simulink model "MPC_Intersection_V2VandAIMandSTL"  (R2021b)
settings: Solver=ode45  StartTime=0.0  StopTime=50  RelTol=1e-3
model workspace (MAT data in the model file):
  firstWarning = 1
  originalScenarioChecksum = '44EB4239245A86A3DA7E3FEB76A9F5A7'
values from neighbouring files (symbols this model uses):
  curvature = (DX.*D2Y - DY.*D2X) ./(DX.^2+DY.^2).^(3/2)    [setUpModel_UScityblock2.m]
  direction = ones(length(gradbp),1)    [setUpModel_UScityblock2.m]
  gradbp = linspace(0,totalDistance,50)    [setUpModel_UScityblock2.m]
  psi_o = thetaRefab(1)*(pi/180)    [setUpModel_UScityblock2.m]
  speed_actor1_gdps = smooth(speedgradbpactor1,speedactor1le)    [velocity_profiles.m]
  speed_actor2_gdps = smooth(speedgradbpactor2,speedactor2le)    [velocity_profiles.m]
  speed_actor3_gdps = smooth(speedgradbpactor3,speedactor3le)    [velocity_profiles.m]
  speed_actor4_gdps = smooth(speedgradbpactor4,speedactor4le)    [velocity_profiles.m]
  speed_ego_gdps = smooth(speedgradbpego,speedegole)    [velocity_profiles.m]
  thetaRefab = zeros(length(gradbp),1)    [setUpModel_UScityblock2.m]
  x_gdps = smooth(gradbp,xwaypoints)    [setUpModel_UScityblock2.m]
  X_o = x_ego_i(1)    [setUpModel_UScityblock2.m]
  y_gdps = smooth(gradbp,ywaypoints)    [setUpModel_UScityblock2.m]
  Y_o = y_ego_i(1)    [setUpModel_UScityblock2.m]
undefined symbols (not defined in the file or in its folder): distancecovered, gradbpA1, gradbpA2, gradbpA3, gradbpA4, gradbpego, magnitude, n, q11, v2xCA
libraries: drivingscenarioandsensors x7, sim3dautolib x5, vehdynlibtirecommon x4, autolibutils x4, aerolibconvert2 x2, mpcadaslib x1, sim3dlib x1, simulink_extras x1, vehdynlibtire x1, simulink x1, autolibshared x1
(part 1 of 2)
settings Model: Creator=REHAN  LastModifiedBy=REHAN

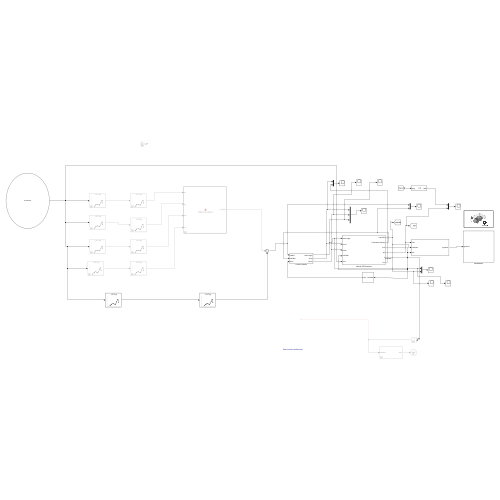
[thumbnail: Simulink's stored preview of the top-level diagram]
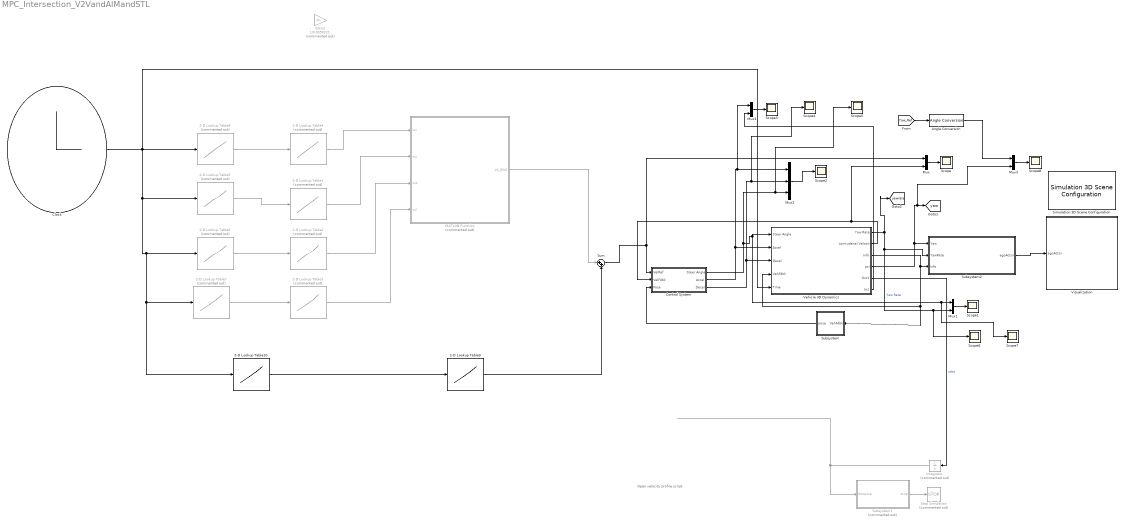
== system MPC_Intersection_V2VandAIMandSTL ==
  note: Open velocity profile script
  2-D Lookup Table1 : Lookup_n-D  Commented=on  NumberOfTableDimensions=1  BreakpointsForDimension1=gradbpA1  BreakpointsForDimension2=q11(:,2)  Table=speed_actor1_gdps  InterpMethod=Cubic spline  InternalRulePriority=Speed  RndMeth=Simplest  InputSameDT=on
  2-D Lookup Table10 : Lookup_n-D  NumberOfTableDimensions=1  BreakpointsForDimension1=n  BreakpointsForDimension2=q11(:,2)  Table=gradbpego  InterpMethod=Cubic spline  InternalRulePriority=Speed  RndMeth=Simplest  InputSameDT=on
  2-D Lookup Table2 : Lookup_n-D  Commented=on  NumberOfTableDimensions=1  BreakpointsForDimension1=gradbpA2  BreakpointsForDimension2=q11(:,2)  Table=speed_actor2_gdps  InterpMethod=Cubic spline  InternalRulePriority=Speed  RndMeth=Simplest  InputSameDT=on
  2-D Lookup Table3 : Lookup_n-D  Commented=on  NumberOfTableDimensions=1  BreakpointsForDimension1=gradbpA3  BreakpointsForDimension2=q11(:,2)  Table=speed_actor3_gdps  InterpMethod=Cubic spline  InternalRulePriority=Speed  RndMeth=Simplest  InputSameDT=on
  2-D Lookup Table4 : Lookup_n-D  Commented=on  NumberOfTableDimensions=1  BreakpointsForDimension1=gradbpA4  BreakpointsForDimension2=q11(:,2)  Table=speed_actor4_gdps  InterpMethod=Cubic spline  InternalRulePriority=Speed  RndMeth=Simplest  InputSameDT=on
  2-D Lookup Table5 : Lookup_n-D  Commented=on  NumberOfTableDimensions=1  BreakpointsForDimension1=n  BreakpointsForDimension2=q11(:,2)  Table=gradbpA1  InterpMethod=Cubic spline  InternalRulePriority=Speed  RndMeth=Simplest  InputSameDT=on
  2-D Lookup Table6 : Lookup_n-D  Commented=on  NumberOfTableDimensions=1  BreakpointsForDimension1=n  BreakpointsForDimension2=q11(:,2)  Table=gradbpA2  InterpMethod=Cubic spline  InternalRulePriority=Speed  RndMeth=Simplest  InputSameDT=on
  2-D Lookup Table7 : Lookup_n-D  Commented=on  NumberOfTableDimensions=1  BreakpointsForDimension1=n  BreakpointsForDimension2=q11(:,2)  Table=gradbpA3  InterpMethod=Cubic spline  InternalRulePriority=Speed  RndMeth=Simplest  InputSameDT=on
  2-D Lookup Table8 : Lookup_n-D  Commented=on  NumberOfTableDimensions=1  BreakpointsForDimension1=n  BreakpointsForDimension2=q11(:,2)  Table=gradbpA4  InterpMethod=Cubic spline  InternalRulePriority=Speed  RndMeth=Simplest  InputSameDT=on
  2-D Lookup Table9 : Lookup_n-D  NumberOfTableDimensions=1  BreakpointsForDimension1=gradbpego  BreakpointsForDimension2=q11(:,2)  Table=v2xCA  InterpMethod=Cubic spline  InternalRulePriority=Speed  RndMeth=Simplest  InputSameDT=on
  Angle Conversion : aerolibconvert2/Angle Conversion  IU=deg  OU=rad
  Clock : Clock
  Control System : Subsystem
  Gain2 : Gain  Commented=on  Gain=1/0.0058221
  Integrator : Integrator  Commented=on  InitialCondition=sqrt((X_o).^2+(Y_o).^2)
  MATLAB Function : MATLAB Function  Commented=on  TreatAsAtomicUnit=on
  Mux{,1,3..4} (4 alike) : Mux  Inputs=2
  Mux2 : Mux  Inputs=3
  Scope{,1..8} (9 alike) : Scope
  Simulation 3D Scene Configuration : sim3dlib/Simulation 3D Scene Configuration  Priority=0  ProjectFormat_internal=Default Scenes  ProjectFormat=Default Scenes  SceneDesc=US city block  ProjectName=C:\Program Files\MATLAB\R2021b\toolbox\shared\sim3d_projects\automotive_project\UE4\WindowsNoEditor\VehicleSimulation.exe  ScenePath=/Game/Maps/HwStrght  vehTagList={'Scene Origin';'SimulinkVehicle1';'SimulinkVehicle2';'SimulinkVehicle3';'SimulinkVehicle4';'SimulinkVehicle5'}  vehTag=SimulinkVehicle1  OpVisEn=off  Ts=1/60  EnableWindow=off  EnableWeather=off  SunAltitude=40.0  SunAzimuth=90  clouds=10  wind=1  fog=0  rain=79.0  sensorTag=MainCamera1  sensorId=1  sensorName=MainCamera1  mountLoc=Origin  offsetFlag=off  tmountOffset=[0, 0, 0]  rmountOffset=[0, 0, 0]  HorizontalResolution=1280  VerticalResolution=720  HorizontalFOV=60  mountPoint=[0 0 0]  mountOrientation=[0 0 0]  aMode=3  ID=1
      settings: SourceProductBaseCode=AE,DR,UV,VE
  Stop Simulation : Stop  Commented=on
  Subsystem : Subsystem
  Subsystem1 : Subsystem  Commented=on
  Subsystem2 : Subsystem
  Sum : Sum  Inputs=|++
  Vehicle 3D Dynamics : Subsystem
  "Visualization " : Subsystem
  tag scope: yaw=global, yawrate=global
  wires:
  Subsystem2/1(egoActor) -> "Visualization "/1(egoActor)
  Vehicle 3D Dynamics/3(Info) -> Subsystem/1(VehFdbk), Vehicle 3D Dynamics/4(VehFdbk), Subsystem2/3(Info)
  Vehicle 3D Dynamics/1(Yaw Rate) -> Scope6/1, Mux1/2, Subsystem2/2(YawRate), [yawrate]  "Yaw Rate"
  Vehicle 3D Dynamics/4(psi) -> Mux3/2, [yaw], Subsystem2/1(Yaw)
  Vehicle 3D Dynamics/2(Lonitudenal Velocity) -> Mux/2, Control System/2(VelFdbk)
  Subsystem/1(pose) -> Control System/3(Pose)
  Control System/2(Accel) -> Mux4/1, Mux2/1, Vehicle 3D Dynamics/2(Accel)
  Control System/3(Decel) -> Scope4/1, Mux2/2, Vehicle 3D Dynamics/3(Decel)
  Mux/1 -> Scope/1
  Mux1/1 -> Scope1/1
  Mux2/1 -> Scope2/1
  [Yaw_Ref] -> Angle Conversion/1
  Mux3/1 -> Scope8/1
  Integrator/1 -> Subsystem1/1(distance)
  Subsystem1/1(stop) -> Stop Simulation/1
  Vehicle 3D Dynamics/5(Out1) -> Integrator/1  "xdot"
  Angle Conversion/1 -> Mux3/1
  Vehicle 3D Dynamics/6(acc) -> Mux4/2
  Mux4/1 -> Scope3/1
  Sum/1 -> Mux/1, Control System/1(VelRef)
  2-D Lookup Table1/1 -> MATLAB Function/2(vxj)
  2-D Lookup Table2/1 -> MATLAB Function/3(vxk)
  2-D Lookup Table3/1 -> MATLAB Function/4(vxl)
  2-D Lookup Table4/1 -> MATLAB Function/1(vxi)
  2-D Lookup Table8/1 -> 2-D Lookup Table4/1
  2-D Lookup Table5/1 -> 2-D Lookup Table1/1
  2-D Lookup Table6/1 -> 2-D Lookup Table2/1
  2-D Lookup Table7/1 -> 2-D Lookup Table3/1
  Clock/1 -> Vehicle 3D Dynamics/5(Time), 2-D Lookup Table10/1, 2-D Lookup Table7/1, 2-D Lookup Table6/1, 2-D Lookup Table5/1, 2-D Lookup Table8/1
  MATLAB Function/1(VX_EGO) -> Sum/1
  2-D Lookup Table10/1 -> 2-D Lookup Table9/1
  2-D Lookup Table9/1 -> Sum/2
  Control System/1(Steer Angle) -> Scope5/1, Mux2/3, Scope7/1, Mux1/1, Vehicle 3D Dynamics/1(Steer Angle)

== system MPC_Intersection_V2VandAIMandSTL/Control System ==
  note: Controller
  VelRef : Inport
  VelFdbk : Inport  Port=2
  Pose : Inport  Port=3
  MPC Based Controller : Subsystem  VariantControl=Stanley
  Steer Angle : Outport
  Accel : Outport  Port=2
  Decel : Outport  Port=3
  wires:
  VelFdbk/1 -> MPC Based Controller/3(VelFdbk)
  Pose/1 -> MPC Based Controller/1(Pose)
  VelRef/1 -> MPC Based Controller/2(VelRef)
  MPC Based Controller/3(DecelCmd) -> Decel/1  "Decel"
  MPC Based Controller/2(AccelCmd) -> Accel/1  "Accel"
  MPC Based Controller/1(WheelSteeringAngle) -> Steer Angle/1  "Steer Angle"

== system MPC_Intersection_V2VandAIMandSTL/Subsystem ==
  VehFdbk : Inport
  Bus Selector : BusSelector  OutputSignals=InertFrm.Cg.Disp.X,InertFrm.Cg.Disp.Y,InertFrm.Cg.Ang.psi
  Gain1 : Gain  Gain=180/pi
  Mux : Mux  Inputs=3
  Transpose : Math  Operator=transpose  SignedPower=on  SaturateOnIntegerOverflow=on
  pose : Outport
  wires:
  Mux/1 -> Transpose/1
  VehFdbk/1 -> Bus Selector/1
  Bus Selector/1 -> Mux/1  "<X>"
  Gain1/1 -> Mux/3
  Bus Selector/2 -> Mux/2  "<Y>"
  Transpose/1 -> pose/1
  Bus Selector/3 -> Gain1/1  "<psi>"

== system MPC_Intersection_V2VandAIMandSTL/Subsystem1 ==
  distance : Inport
  Constant : Constant
  Constant3 : Constant  Value=0
  Switch : Switch  Threshold=distancecovered-10
  stop : Outport
  wires:
  Switch/1 -> stop/1
  Constant3/1 -> Switch/3
  distance/1 -> Switch/2
  Constant/1 -> Switch/1

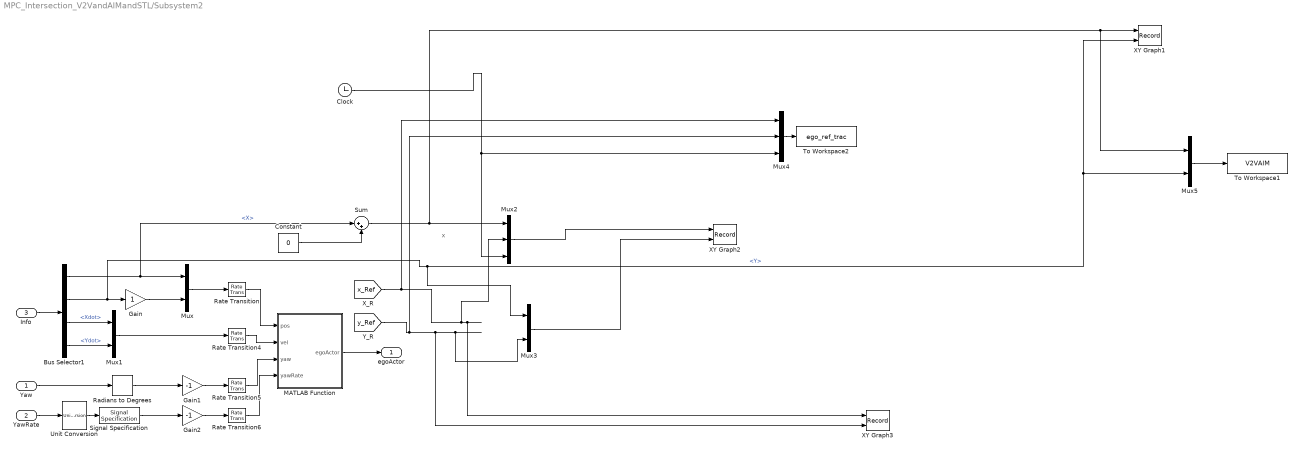
== system MPC_Intersection_V2VandAIMandSTL/Subsystem2 ==
  note: x
  Yaw : Inport
  YawRate : Inport  Port=2
  Info : Inport  Port=3
  Bus Selector1 : BusSelector  OutputSignals=InertFrm.Cg.Disp.X,InertFrm.Cg.Disp.Y,InertFrm.Cg.Vel.Xdot,InertFrm.Cg.Vel.Ydot
  Clock : Clock
  Constant : Constant  Value=0
  Gain : Gain
  Gain1 : Gain  Gain=-1
  Gain2 : Gain  Gain=-1
  MATLAB Function : MATLAB Function  TreatAsAtomicUnit=on
  Mux{,1,3,5} (4 alike) : Mux  Inputs=2
  Mux2 : Mux  Inputs=3
  Mux4 : Mux  Inputs=3
  Radians to Degrees : simulink_extras/Transformations/Radians to Degrees
  Rate Transition{,4..6} (4 alike) : RateTransition
  Signal Specification : SignalSpecification  Unit=deg/s
  Sum : Sum  Inputs=|++
  To Workspace1 : ToWorkspace  VariableName=V2VAIM  SaveFormat=Timeseries  SampleTime=-1
  To Workspace2 : ToWorkspace  VariableName=ego_ref_trac  SaveFormat=Timeseries  SampleTime=-1
  Unit Conversion : UnitConversion
  XY Graph1 : Record  FileSettingsInternal="{\"entries\":[{\"content\":{\"excelSettings\":{\"content\":{},\"type\":\"Streamout.ExcelSettings\"}},\"type\":\"Streamout.FileSettingStorage\",\"uuid\":\"2f12852f-246b-4ef9-8937-bb063900e442\"}],\"packageUris\":[\"http://schema.mathworks.com/mf0/streamout_blocks/R2020a\"],\"version\":\"1.0\"}"  Layout=[1 1]  SignalsInternal="{\"entries\":[{\"content\":{\"signals\":[{\"content\":{\"blockPath\":[\"MPC_Intersection_V2VandAIM/Subsystem2/XY Graph1\"],\"channel\":[],\"dimensions\":[1],\"domain\":\"MPC_Intersection_V2VandAIM/Subsystem2/XY Graph1\",\"lineColor\":\"#d95319\",\"plots\":[],\"port\":1,\"sid\":[\"\"],\"signalID\":357033,\"signalName\":\"Sum\"},\"type\":\"RecordBlkView.Signal\",\"uuid\":\"05f50db8-9dc6-4afe-ab3d-ad6a50919f12\"},{\"content\":{\"blockPath\":[\"MPC_Intersection_V2VandAIM/Subsystem2/XY Graph1\"],\"channel\":[],\"dimensions\":[1],\"domain\":\"MPC_Intersection_V2VandAIM/Subsystem2/XY Graph1\",\"lineColor\":\"#edb120\",\"plots\":[],\"port\":2,\"sid\":[\"\"],\"signalID\":357037,\"signalName\":\"<Y>\"},\"type\":\"RecordBlkView.Signal\",\"uuid\":\"f6264113-20c8-4f22-95b1-a6aed961d63f\"}]},\"type\":\"RecordBlkView.InputSignals\",\"uuid\":\"69c98a76-69b8-42fe-ae6b-722c9eef4afe\"}],\"packageUris\":[\"http://schema.mathworks.com/mf0/streamout_blocks/R2020a\"],\"version\":\"1.0\"}"  VisualizationBindings="{\"xyplotplugin\":{\"info\":[{\"series\":[],\"subplotID\":1}]}}"  CompatibilityTag=XY
  XY Graph2 : Record  FileSettingsInternal="{\"entries\":[{\"content\":{\"excelSettings\":{\"content\":{},\"type\":\"Streamout.ExcelSettings\"}},\"type\":\"Streamout.FileSettingStorage\",\"uuid\":\"6b49d13c-c461-41bf-8846-62c54b908676\"}],\"packageUris\":[\"http://schema.mathworks.com/mf0/streamout_blocks/R2020a\"],\"version\":\"1.0\"}"  Layout=[1 1]  SignalsInternal="{\"entries\":[{\"content\":{\"signals\":[{\"content\":{\"blockPath\":[\"MPC_Intersection_V2VandAIM/Subsystem2/XY Graph2\"],\"channel\":[],\"dimensions\":[3],\"domain\":\"MPC_Intersection_V2VandAIM/Subsystem2/XY Graph2\",\"hasChildren\":true,\"lineColor\":\"#7e2f8e\",\"plots\":[],\"port\":1,\"sid\":[\"\"],\"signalID\":357041,\"signalName\":\"Mux2\"},\"type\":\"RecordBlkView.Signal\",\"uuid\":\"150ad6de-05ca-4e16-9ea5-6f734c90b908\"},{\"content\":{\"blockPath\":[\"MPC_Intersection_V2VandAIM/Subsystem2/XY Graph2\"],\"channel\":[1],\"dimensions\":[3],\"domain\":\"MPC_Intersection_V2VandAIM/Subsystem2/XY Graph2\",\"lineColor\":\"#77ac30\",\"parentID\":357041,\"plots\":[],\"port\":1,\"sid\":[\"\"],\"signalID\":357042,\"signalName\":\"Mux2\"},\"type\":\"RecordBlkView.Signal\",\"uuid\":\"b4915db6-c8af-41c7-9b58-5548bd9cc9e2\"},{\"content\":{\"blockPath\":[\"MPC_Intersection_V2VandAIM/Subsystem2/XY Graph2\"],\"channel\":[],\"dimensions\":[2],\"domain\":\"MPC_Intersection_V2VandAIM/Subsystem2/XY Graph2\",\"hasChildren\":true,\"lineColor\":\"#4dbeee\",\"plots\":[],\"port\":2,\"sid\":[\"\"],\"signalID\":357046,\"signalName\":\"Mux3\"},\"type\":\"RecordBlkView.Signal\",\"uuid\":\"ee75895b-d730-4bf5-9f29-4dbf03fe07c6\"},{\"content\":{\"blockPath\":[\"MPC_Intersection_V2VandAIM/Subsystem2/XY Graph2\"],\"channel\":[1],\"dimensions\":[2],\"domain\":\"MPC_Intersection_V2VandAIM/Subsystem2/XY Graph2\",\"lineColor\":\"#a2142f\",\"parentID\":357046,\"plots\":[],\"port\":2,\"sid\":[\"\"],\"signalID\":357047,\"signalName\":\"Mux3\"},\"type\":\"RecordBlkView.Signal\",\"uuid\":\"339475a3-838f-4545-9489-51cd50d7a86b\"}]},\"type\":\"RecordBlkView.InputSignals\",\"uuid\":\"f0fde65e-7344-42f7-9758-ec72a1af721b\"}],\"packageUris\":[\"http://schema.mathworks.com/mf0/streamout_blocks/R2020a\"],\"version\":\"1.0\"}"  VisualizationBindings="{\"xyplotplugin\":{\"info\":[{\"series\":[],\"subplotID\":1}]}}"  CompatibilityTag=XY
  XY Graph3 : Record  FileSettingsInternal="{\"entries\":[{\"content\":{\"excelSettings\":{\"content\":{},\"type\":\"Streamout.ExcelSettings\"}},\"type\":\"Streamout.FileSettingStorage\",\"uuid\":\"24a241bf-8d8e-474c-b7bc-76b4d2e06980\"}],\"packageUris\":[\"http://schema.mathworks.com/mf0/streamout_blocks/R2020a\"],\"version\":\"1.0\"}"  Layout=[1 1]  SignalsInternal="{\"entries\":[{\"content\":{\"signals\":[{\"content\":{\"blockPath\":[\"MPC_Intersection_V2VandAIM/Subsystem2/XY Graph3\"],\"channel\":[],\"dimensions\":[1],\"domain\":\"MPC_Intersection_V2VandAIM/Subsystem2/XY Graph3\",\"lineColor\":\"#139fff\",\"plots\":[],\"port\":1,\"sid\":[\"\"],\"signalID\":357051,\"signalName\":\"X_R\"},\"type\":\"RecordBlkView.Signal\",\"uuid\":\"67cfc854-4ab1-4cce-b77a-7abc147af39a\"},{\"content\":{\"blockPath\":[\"MPC_Intersection_V2VandAIM/Subsystem2/XY Graph3\"],\"channel\":[],\"dimensions\":[1],\"domain\":\"MPC_Intersection_V2VandAIM/Subsystem2/XY Graph3\",\"lineColor\":\"#ff6929\",\"plots\":[],\"port\":2,\"sid\":[\"\"],\"signalID\":357055,\"signalName\":\"Y_R\"},\"type\":\"RecordBlkView.Signal\",\"uuid\":\"aa72a502-d578-4dc8-aeef-fdcf7ff26e0e\"}]},\"type\":\"RecordBlkView.InputSignals\",\"uuid\":\"33211d98-26d3-424d-a838-ac910746517b\"}],\"packageUris\":[\"http://schema.mathworks.com/mf0/streamout_blocks/R2020a\"],\"version\":\"1.0\"}"  VisualizationBindings="{\"xyplotplugin\":{\"info\":[{\"series\":[],\"subplotID\":1}]}}"  CompatibilityTag=XY
  egoActor : Outport
  wires:
  Mux/1 -> Rate Transition/1
  Rate Transition/1 -> MATLAB Function/1(pos)
  Rate Transition4/1 -> MATLAB Function/2(vel)
  Signal Specification/1 -> Gain2/1
  Bus Selector1/4 -> Mux1/2  "<Ydot>"
  Rate Transition5/1 -> MATLAB Function/3(yaw)
  Rate Transition6/1 -> MATLAB Function/4(yawRate)
  Bus Selector1/1 -> Sum/1, Mux/1  "<X>"
  Mux1/1 -> Rate Transition4/1
  YawRate/1 -> Unit Conversion/1
  Yaw/1 -> Radians to Degrees/1
  Radians to Degrees/1 -> Gain1/1
  Info/1 -> Bus Selector1/1
  Gain2/1 -> Rate Transition6/1
  Unit Conversion/1 -> Signal Specification/1
  Gain1/1 -> Rate Transition5/1
  Bus Selector1/3 -> Mux1/1  "<Xdot>"
  MATLAB Function/1(egoActor) -> egoActor/1
  [x_Ref] -> Mux4/1, Mux2/2, XY Graph3/1
  Gain/1 -> Mux/2
  [y_Ref] -> Mux4/2, XY Graph3/2, Mux3/2
  Mux2/1 -> XY Graph2/1
  Mux3/1 -> XY Graph2/2
  Bus Selector1/2 -> Mux3/1, XY Graph1/2, Mux5/2, Gain/1  "<Y>"
  Sum/1 -> XY Graph1/1, Mux5/1, Mux2/1
  Constant/1 -> Sum/2
  Clock/1 -> Mux4/3, Mux2/3
  Mux5/1 -> To Workspace1/1
  Mux4/1 -> To Workspace2/1

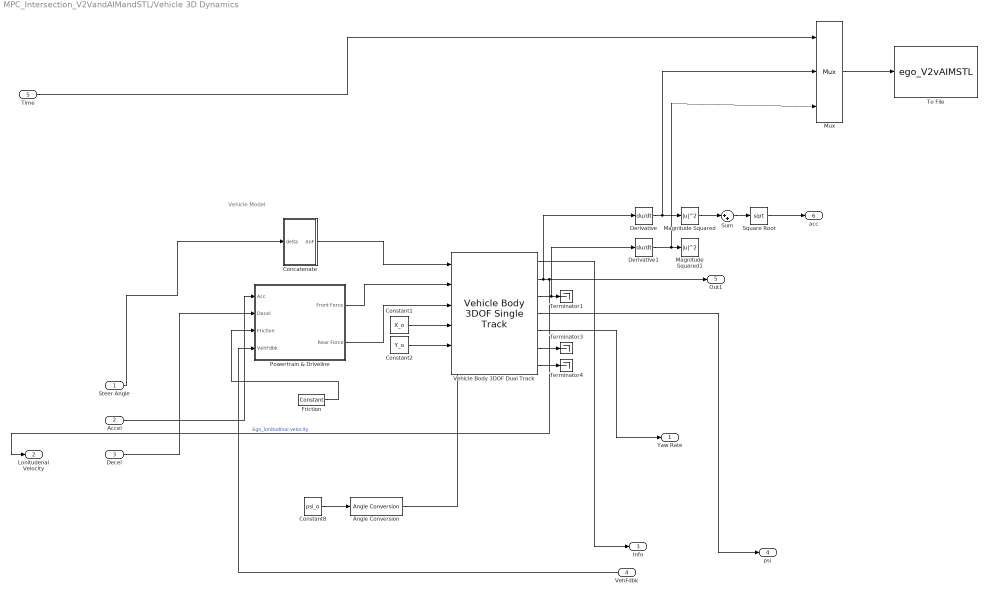
== system MPC_Intersection_V2VandAIMandSTL/Vehicle 3D Dynamics ==
  note: Vehicle Model
  Steer Angle : Inport
  Accel : Inport  Port=2
  Decel : Inport  Port=3
  VehFdbk : Inport  Port=4
  Time : Inport  Port=5
  Angle Conversion : aerolibconvert2/Angle Conversion  IU=rad  OU=deg
  Concatenate : Subsystem
  Constant1 : Constant  Value=X_o
  Constant2 : Constant  Value=Y_o
  Constant8 : Constant  Value=psi_o
  Derivative : Derivative
  Derivative1 : Derivative
  Friction : vehdynlibtirecommon/Constant  const=1  numWheels=4
      settings: SourceProductBaseCode=VE
  Magnitude Squared : Math  Operator=magnitude^2  SaturateOnIntegerOverflow=on
  Magnitude Squared1 : Math  Operator=magnitude^2  SaturateOnIntegerOverflow=on
  Mux : Mux  Inputs=3
  Powertrain & Driveline : Subsystem
      mask Display: image('vdbslibpt.png');
  Square Root : Sqrt  SaturateOnIntegerOverflow=on
  Sum : Sum  Inputs=|++
  Terminator1 : Terminator
  Terminator3 : Terminator
  Terminator4 : Terminator
  To File : ToFile  Filename=ego_V2vAIMSTL  MatrixName=waypointstimeseries
      settings: Decimation=100
  Vehicle Body 3DOF Dual Track : autolibshared/Vehicle Body 3DOF Single Track  trackMode=Dual  inputMode=External forces  frontSteerMode=on  rearSteerMode=off  windMode=off  muMode=off  extFMode=off  extMMode=off  htchFMode=off  htchMMode=off  extXo=on  extpsio=on  extxdoto=off  extro=off  extYo=on  extTamb=off  extydoto=off  aMode=2  NF=2  NR=2  m=2000  a=1.4  b=1.4  h=0.35  dh=1  hh=0.2  X_o=0  xdot_o=speed_ego_gdps(1)  CalphaMode=off  sigmaMode=on  d=0  hl=0  w=[1.4,1.4]  Cy_f=12e3  Cy_r=11e3  sigma_f=.1  sigma_r=.1  alpha_f_brk=[-.1 .1]  Cy_f_data=[-9e3 9e3]  alpha_r_brk=[-.1 .1]  Cy_r_data=[-9e3 9e3]  Y_o=0  ydot_o=0  Izz=1000  psi_o=0  r_o=0  Af=2  Cd=.3  Cl=.1  Cpm=.1  beta_w=[0:0.01:0.3]  Cs=[0:0.03:0.9]  Cym=[0:0.01:0.3]  Pabs=101325  Tair=273  g=9.81  mu=1  xdot_tol=.01  Fznom=5000  Fxtire_sat=7e4  Fytire_sat=7e4  longOff=0  latOff=0  vertOff=0  wrapAng=off
      settings: SourceProductBaseCode=PW,DR,MT,UV,VE
  Yaw Rate : Outport
  Lonitudenal Velocity : Outport  Port=2
  Info : Outport  Port=3
  psi : Outport  Port=4
  Out1 : Outport  Port=5
  acc : Outport  Port=6
  wires:
  Decel/1 -> Powertrain & Driveline/2(Decel)
  Constant8/1 -> Angle Conversion/1
  Vehicle Body 3DOF Dual Track/7 -> Terminator4/1
  Vehicle Body 3DOF Dual Track/1 -> Info/1
  Vehicle Body 3DOF Dual Track/6 -> Terminator3/1
  Constant2/1 -> Vehicle Body 3DOF Dual Track/5
  Friction/1 -> Powertrain & Driveline/3(Friction)
  Vehicle Body 3DOF Dual Track/2 -> Derivative/1, Out1/1, Lonitudenal Velocity/1  "Ego_lonitudinal velocity"
  Vehicle Body 3DOF Dual Track/3 -> Derivative1/1, Terminator1/1
  Constant1/1 -> Vehicle Body 3DOF Dual Track/4
  Accel/1 -> Powertrain & Driveline/1(Acc)
  Vehicle Body 3DOF Dual Track/5 -> Yaw Rate/1
  Vehicle Body 3DOF Dual Track/4 -> psi/1
  VehFdbk/1 -> Powertrain & Driveline/4(VehFdbk)
  Steer Angle/1 -> Concatenate/1(delta)
  Concatenate/1(AnF) -> Vehicle Body 3DOF Dual Track/1
  Angle Conversion/1 -> Vehicle Body 3DOF Dual Track/6
  Derivative/1 -> Mux/2, Magnitude Squared/1
  Derivative1/1 -> Mux/3, Magnitude Squared1/1
  Magnitude Squared/1 -> Sum/1
  Sum/1 -> Square Root/1
  Square Root/1 -> acc/1
  Time/1 -> Mux/1
  Mux/1 -> To File/1
  Powertrain & Driveline/1(Front Force) -> Vehicle Body 3DOF Dual Track/2
  Powertrain & Driveline/2(Rear Force) -> Vehicle Body 3DOF Dual Track/3

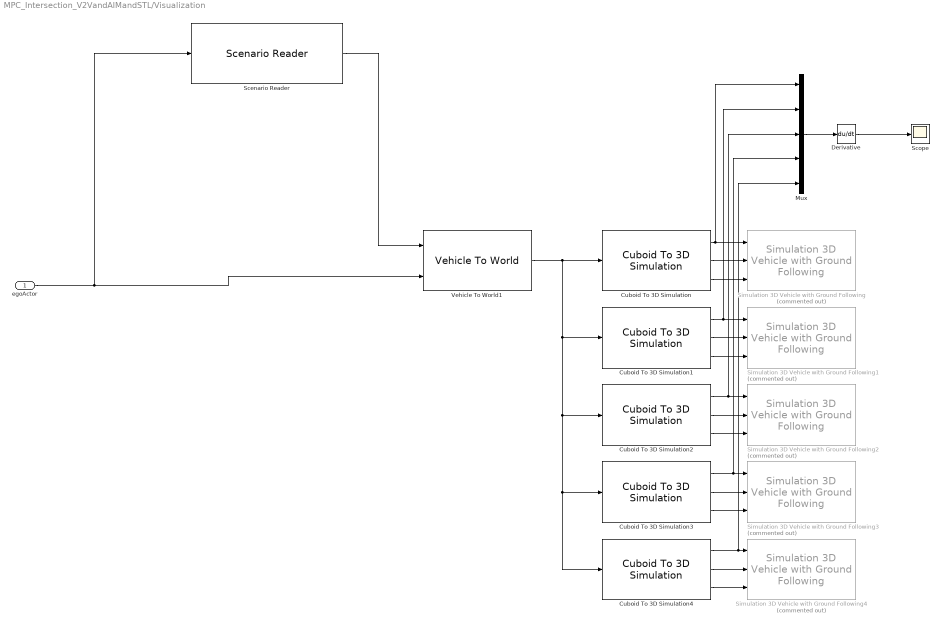
== system MPC_Intersection_V2VandAIMandSTL/Visualization  ==
  egoActor : Inport
  Cuboid To 3D Simulation : drivingscenarioandsensors/Cuboid To 3D Simulation  SpecifyActorID=off  ActorIDToConvert=1  SimulateUsing=Interpreted execution
      settings: SourceProductBaseCode=DR
  Cuboid To 3D Simulation1 : drivingscenarioandsensors/Cuboid To 3D Simulation  SpecifyActorID=off  ActorIDToConvert=2  SimulateUsing=Interpreted execution
      settings: SourceProductBaseCode=DR
  Cuboid To 3D Simulation2 : drivingscenarioandsensors/Cuboid To 3D Simulation  SpecifyActorID=off  ActorIDToConvert=3  SimulateUsing=Interpreted execution
      settings: SourceProductBaseCode=DR
  Cuboid To 3D Simulation3 : drivingscenarioandsensors/Cuboid To 3D Simulation  SpecifyActorID=off  ActorIDToConvert=4  SimulateUsing=Interpreted execution
      settings: SourceProductBaseCode=DR
  Cuboid To 3D Simulation4 : drivingscenarioandsensors/Cuboid To 3D Simulation  SpecifyActorID=off  ActorIDToConvert=4  SimulateUsing=Interpreted execution
      settings: SourceProductBaseCode=DR
  Derivative : Derivative
  Mux : Mux  Inputs=5
  Scenario Reader : drivingscenarioandsensors/Scenario Reader  ScenarioSource=From file  ScenarioFileName=C:\Users\REHAN\OneDrive - The Ohio State University\UTC PNT Resilience\simulation files\USCityBlock2.mat  ScenarioVariableName=scenario  OutputCoordinateSystem=Vehicle coordinates  EgoVehicleSource=Input port  EgoVehicleActorID=1  OrientVehiclesOnRoad=on  OutputEgoVehiclePose=on  OutputEgoVehicleState=off  SampleTime=0.1  LaneBoundaryOutput=None  LaneBoundaryDistance=0:0.5:9.5  LaneBoundaryLocation=Center of lane markings  BusNameSource=Auto  BusName=BusActors  BusNumActorsSource=Scenario  BusNumActors=100  BusName2Source=Auto  BusName2=BusLaneBoundaries  BusNumLaneBoundariesSource=Scenario  BusNumLaneBoundaries=10  BusName3Source=Auto  BusName3=BusEgoActor  BusName4Source=Auto  BusName4=BusEgoState  ShowCoordinateLabels=on  SimulateUsing=Interpreted execution
  Scope : Scope
  Simulation 3D Vehicle with Ground Following : sim3dautolib/Simulation 3D Vehicle with Ground Following  Priority=-1  Commented=on  PassVehMesh=Muscle car  PassVehMesh_Internal=Muscle car  MeshPath=/MathWorksSimulation/Vehicles/Muscle/Meshes/SK_MuscleCar.SK_MuscleCar  TrackWidth=1.9  WheelBase=3  WheelRadius=0.35  VehColor=Red  VehColor_Internal=Red  InitialPos=[-150.9000,-1.8000, 0]  InitialRot=[0, 0,0.6853]  ActorName=SimulinkVehicle1  SampleTime=-1  ActorType=SimulinkVehicle  ID=1  aMode=3  ActorTag=SimulinkVehicle1  CoordinateScheme=ISO  VehLightsControl=off  HeadlightColor=[ 1, 1, 1 ]  HighBeamIntensity=100000  LowBeamIntensity=60000  HighBeamConeAngle=70  LowBeamConeAngle=70  LeftHeadlightOrientation=[ 0, 0 ]  RightHeadlightOrientation=[ 0, 0 ]  BrakelightIntensity=500  ReverselightIntensity=500  SignallightIntensity=500  SignallightPeriod=1  SignalPulseWidth=50  TransformOutportEnabled=off
      settings: SourceProductBaseCode=AE,DR,UV,VE
  Simulation 3D Vehicle with Ground Following1 : sim3dautolib/Simulation 3D Vehicle with Ground Following  Priority=-1  Commented=on  PassVehMesh=Muscle car  PassVehMesh_Internal=Muscle car  MeshPath=/MathWorksSimulation/Vehicles/Muscle/Meshes/SK_MuscleCar.SK_MuscleCar  TrackWidth=1.9  WheelBase=3  WheelRadius=0.35  VehColor=Orange  VehColor_Internal=Orange  InitialPos=[-110.9713, -28.0022, 0]  InitialRot=[0, 0, 86.1785]  ActorName=SimulinkVehicle2  SampleTime=-1  ActorType=SimulinkVehicle  ID=2  aMode=3  ActorTag=SimulinkVehicle2  CoordinateScheme=ISO  VehLightsControl=off  HeadlightColor=[ 1, 1, 1 ]  HighBeamIntensity=100000  LowBeamIntensity=60000  HighBeamConeAngle=70  LowBeamConeAngle=70  LeftHeadlightOrientation=[ 0, 0 ]  RightHeadlightOrientation=[ 0, 0 ]  BrakelightIntensity=500  ReverselightIntensity=500  SignallightIntensity=500  SignallightPeriod=1  SignalPulseWidth=50  TransformOutportEnabled=off
      settings: SourceProductBaseCode=AE,DR,UV,VE
  Simulation 3D Vehicle with Ground Following2 : sim3dautolib/Simulation 3D Vehicle with Ground Following  Priority=-1  Commented=on  PassVehMesh=Muscle car  PassVehMesh_Internal=Muscle car  MeshPath=/MathWorksSimulation/Vehicles/Muscle/Meshes/SK_MuscleCar.SK_MuscleCar  TrackWidth=1.9  WheelBase=3  WheelRadius=0.35  VehColor=Green  VehColor_Internal=Green  InitialPos=[-84.2000, 2.50, 0]  InitialRot=[0, 0, 176.7404]  ActorName=SimulinkVehicle3  SampleTime=-1  ActorType=SimulinkVehicle  ID=3  aMode=3  ActorTag=SimulinkVehicle3  CoordinateScheme=ISO  VehLightsControl=off  HeadlightColor=[ 1, 1, 1 ]  HighBeamIntensity=100000  LowBeamIntensity=60000  HighBeamConeAngle=70  LowBeamConeAngle=70  LeftHeadlightOrientation=[ 0, 0 ]  RightHeadlightOrientation=[ 0, 0 ]  BrakelightIntensity=500  ReverselightIntensity=500  SignallightIntensity=500  SignallightPeriod=1  SignalPulseWidth=50  TransformOutportEnabled=off
      settings: SourceProductBaseCode=AE,DR,UV,VE
  Simulation 3D Vehicle with Ground Following3 : sim3dautolib/Simulation 3D Vehicle with Ground Following  Priority=-1  Commented=on  PassVehMesh=Muscle car  PassVehMesh_Internal=Muscle car  MeshPath=/MathWorksSimulation/Vehicles/Muscle/Meshes/SK_MuscleCar.SK_MuscleCar  TrackWidth=1.9  WheelBase=3  WheelRadius=0.35  VehColor=Blue  VehColor_Internal=Blue  InitialPos=[-114.9284, 33.7974, 0]  InitialRot=[0, 0, 84.2930]  ActorName=SimulinkVehicle4  SampleTime=-1  ActorType=SimulinkVehicle  ID=4  aMode=3  ActorTag=SimulinkVehicle4  CoordinateScheme=ISO  VehLightsControl=off  HeadlightColor=[ 1, 1, 1 ]  HighBeamIntensity=100000  LowBeamIntensity=60000  HighBeamConeAngle=70  LowBeamConeAngle=70  LeftHeadlightOrientation=[ 0, 0 ]  RightHeadlightOrientation=[ 0, 0 ]  BrakelightIntensity=500  ReverselightIntensity=500  SignallightIntensity=500  SignallightPeriod=1  SignalPulseWidth=50  TransformOutportEnabled=off
      settings: SourceProductBaseCode=AE,DR,UV,VE
  Simulation 3D Vehicle with Ground Following4 : sim3dautolib/Simulation 3D Vehicle with Ground Following  Priority=-1  Commented=on  PassVehMesh=Muscle car  PassVehMesh_Internal=Muscle car  MeshPath=/MathWorksSimulation/Vehicles/Muscle/Meshes/SK_MuscleCar.SK_MuscleCar  TrackWidth=1.9  WheelBase=3  WheelRadius=0.35  VehColor=Red  VehColor_Internal=Red  InitialPos=[X_o, Y_o, 0]  InitialRot=[0, 0, psi_o]  ActorName=SimulinkVehicle5  SampleTime=-1  ActorType=SimulinkVehicle  ID=5  aMode=3  ActorTag=SimulinkVehicle5  CoordinateScheme=ISO  VehLightsControl=off  HeadlightColor=[ 1, 1, 1 ]  HighBeamIntensity=100000  LowBeamIntensity=60000  HighBeamConeAngle=70  LowBeamConeAngle=70  LeftHeadlightOrientation=[ 0, 0 ]  RightHeadlightOrientation=[ 0, 0 ]  BrakelightIntensity=500  ReverselightIntensity=500  SignallightIntensity=500  SignallightPeriod=1  SignalPulseWidth=50  TransformOutportEnabled=off
      settings: SourceProductBaseCode=AE,DR,UV,VE
  Vehicle To World1 : drivingscenarioandsensors/Vehicle To World  BusNameSource=Auto  BusName=BusVehicleToWorldActors  SimulateUsing=Interpreted execution
      settings: SourceProductBaseCode=DR
  wires:
  Cuboid To 3D Simulation2/3 -> Simulation 3D Vehicle with Ground Following2/3
  Cuboid To 3D Simulation/3 -> Simulation 3D Vehicle with Ground Following/3
  Vehicle To World1/1 -> Cuboid To 3D Simulation4/1, Cuboid To 3D Simulation3/1, Cuboid To 3D Simulation2/1, Cuboid To 3D Simulation1/1, Cuboid To 3D Simulation/1
  Cuboid To 3D Simulation2/1 -> Mux/3, Simulation 3D Vehicle with Ground Following2/1
  Cuboid To 3D Simulation/2 -> Simulation 3D Vehicle with Ground Following/2
  Cuboid To 3D Simulation/1 -> Mux/1, Simulation 3D Vehicle with Ground Following/1
  Cuboid To 3D Simulation2/2 -> Simulation 3D Vehicle with Ground Following2/2
  Cuboid To 3D Simulation3/2 -> Simulation 3D Vehicle with Ground Following3/2
  Cuboid To 3D Simulation3/1 -> Mux/4, Simulation 3D Vehicle with Ground Following3/1
  Cuboid To 3D Simulation3/3 -> Simulation 3D Vehicle with Ground Following3/3
  Cuboid To 3D Simulation1/3 -> Simulation 3D Vehicle with Ground Following1/3
  Cuboid To 3D Simulation1/1 -> Mux/2, Simulation 3D Vehicle with Ground Following1/1
  Cuboid To 3D Simulation1/2 -> Simulation 3D Vehicle with Ground Following1/2
  Cuboid To 3D Simulation4/1 -> Mux/5, Simulation 3D Vehicle with Ground Following4/1
  Cuboid To 3D Simulation4/2 -> Simulation 3D Vehicle with Ground Following4/2
  Cuboid To 3D Simulation4/3 -> Simulation 3D Vehicle with Ground Following4/3
  Scenario Reader/1 -> Vehicle To World1/1
  egoActor/1 -> Scenario Reader/1, Vehicle To World1/2
  Derivative/1 -> Scope/1
  Mux/1 -> Derivative/1

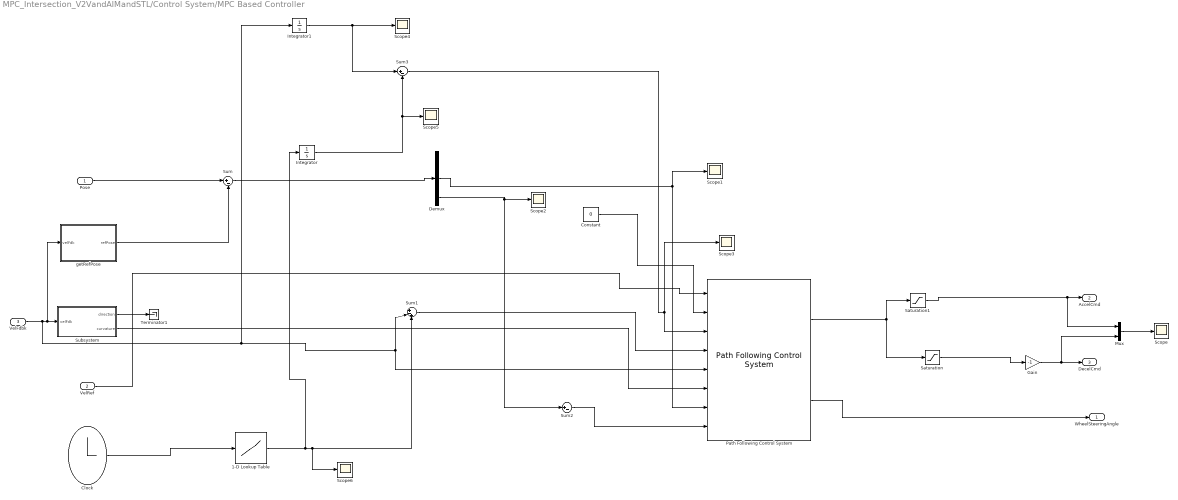
== system MPC_Intersection_V2VandAIMandSTL/Control System/MPC Based Controller ==
  Pose : Inport
  VelRef : Inport  Port=2
  VelFdbk : Inport  Port=3
  1-D Lookup Table : Lookup_n-D  NumberOfTableDimensions=1  BreakpointsForDimension1=n  Table=speed_actor4_gdps  InternalRulePriority=Speed  RndMeth=Simplest  InputSameDT=on
  Clock : Clock
  Constant : Constant  Value=0
  Demux : Demux  Outputs=3
  Gain : Gain  Gain=-1
  Integrator : Integrator
  Integrator1 : Integrator
  Mux : Mux  Inputs=2
  Path Following Control System : mpcadaslib/Path Following Control System  VariantControl=Variant2  ModelType=Use vehicle parameters  VehicleMass=1575  VehicleYawInertia=2875  LengthToFront=1.2  LengthToRear=1.6  FrontTireStiffness=19000  RearTireStiffness=33000  AccelTimeConstant=0.5  EgoModelMatrixA=[-2,zeros(1,3);1,zeros(1,3);zeros(1,2),-4.4021,-12.4603;zeros(1,2),1.3913,-5.1868]  EgoModelMatrixB=[2,zeros(1,3);zeros(1,2),24.1270,15.8609]'  EgoModelMatrixC=[zeros(3,1),eye(3)]  InitialLongVel=1  TransportLag=0  spaceCtrl=on  DefaultSpacing=0  MinSteering=-0.86  umin_ext=off  MaxSteering=0.86  umax_ext=off  MinAcceleration=-0.86  amin_ext=off  MaxAcceleration=0.86  amax_ext=off  Ts=0.1  PredictionHorizon=50  ControlHorizon=2  LongWeight=5000  LateralWeight=0.01  AccelRateWeight=3  SteerRateWeight=20  suboptimal=off  maxiter=10  datatypeopt=double  optmode=off  trackmode=off
      settings: SourceProductBaseCode=MP
  Saturation : Saturate  UpperLimit=0  LowerLimit=-3
  Saturation1 : Saturate  UpperLimit=3  LowerLimit=0
  Scope{,1..6} (7 alike) : Scope
  Subsystem : Subsystem
  Sum : Sum  Inputs=|+-
  Sum1 : Sum  Inputs=|+-+
  Sum2 : Sum  Inputs=|+-
  Sum3 : Sum  Inputs=|+-
  Terminator1 : Terminator
  getRefPose : Subsystem
  WheelSteeringAngle : Outport
  AccelCmd : Outport  Port=2
  DecelCmd : Outport  Port=3
  wires:
  VelFdbk/1 -> Integrator1/1, Path Following Control System/5, Sum1/2, Subsystem/1(velFdk), getRefPose/1(velFdk)
  getRefPose/1(refPose) -> Sum/2
  Subsystem/2(curvature) -> Path Following Control System/6
  Constant/1 -> Path Following Control System/2
  Path Following Control System/2 -> WheelSteeringAngle/1
  Path Following Control System/1 -> Saturation1/1, Saturation/1
  Saturation/1 -> Gain/1
  Mux/1 -> Scope/1
  Gain/1 -> Mux/2, DecelCmd/1
  Demux/2 -> Scope1/1, Path Following Control System/7
  Pose/1 -> Sum/1
  Subsystem/1(direction) -> Terminator1/1
  Saturation1/1 -> Mux/1, AccelCmd/1
  Sum/1 -> Demux/1
  Sum1/1 -> Path Following Control System/4
  Sum2/1 -> Path Following Control System/8
  Demux/3 -> Scope2/1, Sum2/1
  1-D Lookup Table/1 -> Integrator/1, Scope6/1, Sum1/3
  Clock/1 -> 1-D Lookup Table/1
  Sum3/1 -> Scope3/1, Path Following Control System/3
  Integrator1/1 -> Scope4/1, Sum3/1
  Integrator/1 -> Scope5/1, Sum3/2
  VelRef/1 -> Path Following Control System/1

== system MPC_Intersection_V2VandAIMandSTL/Vehicle 3D Dynamics/Concatenate ==
  delta : Inport
  Matrix Concatenate : Concatenate
  AnF : Outport  VectorParamsAs1DForOutWhenUnconnected=off
  tag scope: AnL=global, AnR=global
  wires:
  Matrix Concatenate/1 -> AnF/1
  delta/1 -> [AnR], Matrix Concatenate/2, Matrix Concatenate/1, [AnL]

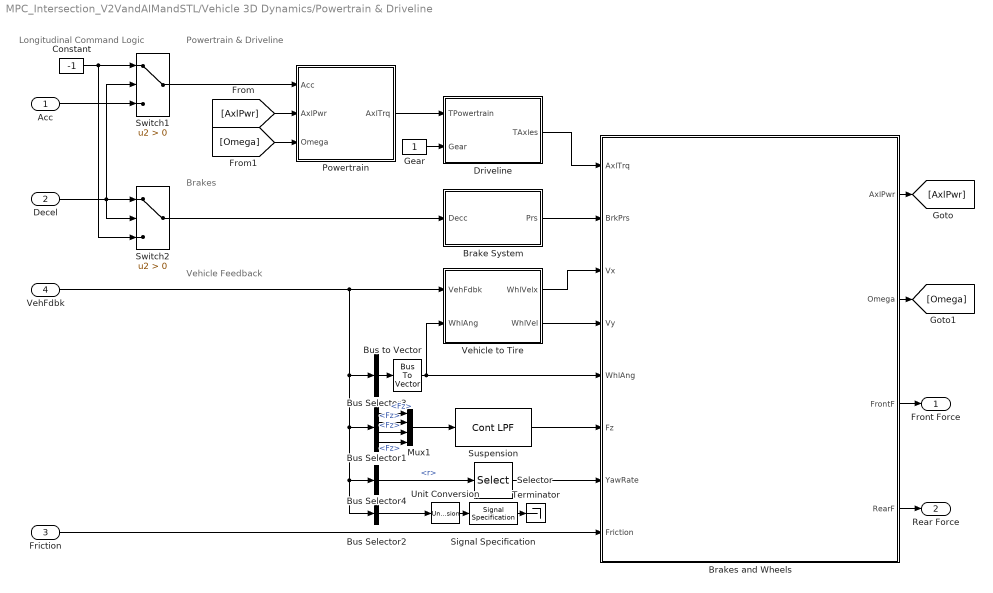
== system MPC_Intersection_V2VandAIMandSTL/Vehicle 3D Dynamics/Powertrain & Driveline ==
  note: Vehicle Feedback
  note: Powertrain & Driveline
  note: Brakes
  note: Longitudinal Command Logic
  Acc : Inport
  Decel : Inport  Port=2
  Friction : Inport  Port=3
  VehFdbk : Inport  Port=4
  Brake System : Subsystem
  Brakes and Wheels : Subsystem  TreatAsAtomicUnit=on
      mask Display: image('vdbslibwhls.png');
  Bus Selector1 : BusSelector  OutputSignals=BdyFrm.Forces.Tires.FrntTires.Lft.Fz,BdyFrm.Forces.Tires.FrntTires.Rght.Fz,BdyFrm.Forces.Tires.RearTires.Lft.Fz,BdyFrm.Forces.Tires.RearTires.Rght.Fz
  Bus Selector2 : BusSelector  OutputSignals=BdyFrm.Cg.Vel.xdot  OutputAsBus=on
  Bus Selector3 : BusSelector  OutputSignals=BdyFrm.FrntAxl.Steer.WhlAngFL,BdyFrm.FrntAxl.Steer.WhlAngFR,BdyFrm.RearAxl.Steer.WhlAngRL,BdyFrm.RearAxl.Steer.WhlAngRR  OutputAsBus=on
  Bus Selector4 : BusSelector  OutputSignals=BdyFrm.Cg.AngVel.r
  Bus to Vector : BusToVector
  Constant : Constant  Value=-1
  Driveline : Subsystem  Variant=on  VariantControlMode=label  VariantControl=Variant1  LabelModeActiveChoice=0
  Gear : Constant
  Mux1 : Mux
  Powertrain : Subsystem
  Selector : Selector  InputPortWidth=1  IndexOptions=Index vector (dialog)  Indices=[1 1 1 1]  OutputSizes=1
  Signal Specification : SignalSpecification  Unit=km/hr
  Suspension : autolibutils/Cont LPF  wc=10*pi*2  aMode=2
      settings: SourceProductBaseCode=PW,DR,MT,UV,VE
  Switch1 : Switch  Criteria=u2 > Threshold
  Switch2 : Switch  Criteria=u2 > Threshold
  Terminator : Terminator
  Unit Conversion : UnitConversion
  Vehicle to Tire : Subsystem
  Front Force : Outport  VectorParamsAs1DForOutWhenUnconnected=off
  Rear Force : Outport  Port=2  VectorParamsAs1DForOutWhenUnconnected=off
  wires:
  Vehicle to Tire/2(WhlVel) -> Brakes and Wheels/4(Vy)
  Vehicle to Tire/1(WhlVelx) -> Brakes and Wheels/3(Vx)
  Brakes and Wheels/1(AxlPwr) -> [AxlPwr]
  Brakes and Wheels/4(RearF) -> Rear Force/1
  Brakes and Wheels/3(FrontF) -> Front Force/1
  Brakes and Wheels/2(Omega) -> [Omega]
  VehFdbk/1 -> Vehicle to Tire/1(VehFdbk), Bus Selector3/1, Bus Selector1/1, Bus Selector4/1, Bus Selector2/1
  Selector/1 -> Brakes and Wheels/7(YawRate)
  Bus Selector4/1 -> Selector/1  "<r>"
  Friction/1 -> Brakes and Wheels/8(Friction)
  Gear/1 -> Driveline/2(Gear)
  Signal Specification/1 -> Terminator/1
  Unit Conversion/1 -> Signal Specification/1
  Bus Selector2/1 -> Unit Conversion/1
  Brake System/1(Prs) -> Brakes and Wheels/2(BrkPrs)
  Switch2/1 -> Brake System/1(Decc)
  [Omega] -> Powertrain/3(Omega)
  [AxlPwr] -> Powertrain/2(AxlPwr)
  Powertrain/1(AxlTrq) -> Driveline/1(TPowertrain)
  Switch1/1 -> Powertrain/1(Acc)
  Bus Selector1/4 -> Mux1/4  "<Fz>"
  Bus Selector1/3 -> Mux1/3  "<Fz>"
  Bus Selector1/2 -> Mux1/2  "<Fz>"
  Bus Selector1/1 -> Mux1/1  "<Fz>"
  Suspension/1 -> Brakes and Wheels/6(Fz)
  Mux1/1 -> Suspension/1
  Bus to Vector/1 -> Brakes and Wheels/5(WhlAng), Vehicle to Tire/2(WhlAng)
  Bus Selector3/1 -> Bus to Vector/1
  Driveline/1(TAxles) -> Brakes and Wheels/1(AxlTrq)
  Constant/1 -> Switch1/1, Switch2/3
  Acc/1 -> Switch1/3
  Decel/1 -> Switch2/1, Switch2/2, Switch1/2

== system MPC_Intersection_V2VandAIMandSTL/Control System/MPC Based Controller/Subsystem ==
  velFdk : Inport
  Curvature : Lookup_n-D  NumberOfTableDimensions=1  BreakpointsForDimension1=gradbp  Table=curvature  InternalRulePriority=Speed  RndMeth=Simplest  InputSameDT=on
  Direction : Lookup_n-D  NumberOfTableDimensions=1  BreakpointsForDimension1=gradbp  Table=direction  InternalRulePriority=Speed  RndMeth=Simplest  InputSameDT=on
  Integrator1 : Integrator
  direction : Outport
  curvature : Outport  Port=2
  wires:
  velFdk/1 -> Integrator1/1
  Integrator1/1 -> Direction/1, Curvature/1
  Curvature/1 -> curvature/1
  Direction/1 -> direction/1

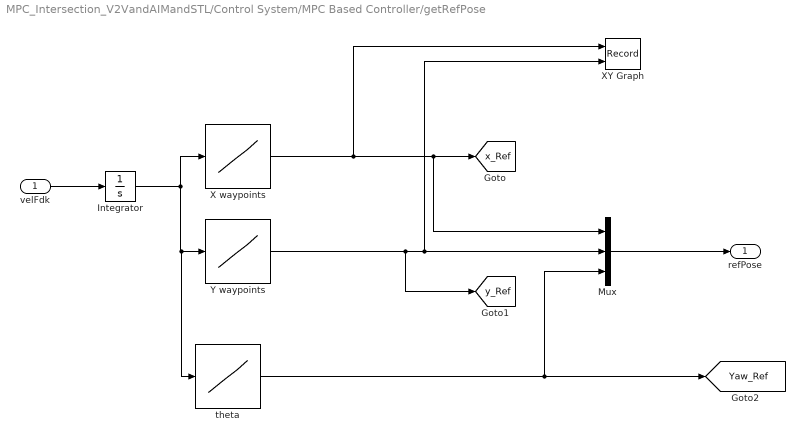
== system MPC_Intersection_V2VandAIMandSTL/Control System/MPC Based Controller/getRefPose ==
  velFdk : Inport
  Integrator : Integrator
  Mux : Mux  Inputs=3
  X waypoints : Lookup_n-D  NumberOfTableDimensions=1  BreakpointsForDimension1=gradbp  Table=x_gdps  InternalRulePriority=Speed  RndMeth=Simplest  InputSameDT=on
  XY Graph : Record  FileSettingsInternal="{\"entries\":[{\"content\":{\"excelSettings\":{\"content\":{},\"type\":\"Streamout.ExcelSettings\"}},\"type\":\"Streamout.FileSettingStorage\",\"uuid\":\"6aa8ae91-f7ce-496f-92bb-696a5a705436\"}],\"packageUris\":[\"http://schema.mathworks.com/mf0/streamout_blocks/R2020a\"],\"version\":\"1.0\"}"  Layout=[1 1]  SignalsInternal="{\"entries\":[{\"content\":{\"signals\":[{\"content\":{\"blockPath\":[\"MPC_Intersection_V2VandAIM/Control System/MPC Based Controller/getRefPose/XY Graph\"],\"channel\":[],\"dimensions\":[1],\"domain\":\"MPC_Intersection_V2VandAIM/Control System/MPC Based Controller/getRefPose/XY Graph\",\"lineColor\":\"#22b573\",\"plots\":[],\"port\":1,\"sid\":[\"\"],\"signalID\":357025,\"signalName\":\"X waypoints\"},\"type\":\"RecordBlkView.Signal\",\"uuid\":\"165d2a0c-33ff-47a3-a9f6-a99102be3ac1\"},{\"content\":{\"blockPath\":[\"MPC_Intersection_V2VandAIM/Control System/MPC Based Controller/getRefPose/XY Graph\"],\"channel\":[],\"dimensions\":[1],\"domain\":\"MPC_Intersection_V2VandAIM/Control System/MPC Based Controller/getRefPose/XY Graph\",\"lineColor\":\"#0072bd\",\"plots\":[],\"port\":2,\"sid\":[\"\"],\"signalID\":357029,\"signalName\":\"Y waypoints\"},\"type\":\"RecordBlkView.Signal\",\"uuid\":\"55140c9b-f205-4a31-9971-9d327590276e\"}]},\"type\":\"RecordBlkView.InputSignals\",\"uuid\":\"8cef2a80-f974-474f-9630-9d0ec5a192ec\"}],\"packageUris\":[\"http://schema.mathworks.com/mf0/streamout_blocks/R2020a\"],\"version\":\"1.0\"}"  VisualizationBindings="{\"xyplotplugin\":{\"info\":[{\"series\":[],\"subplotID\":1}]}}"  CompatibilityTag=XY
  Y waypoints : Lookup_n-D  NumberOfTableDimensions=1  BreakpointsForDimension1=gradbp  Table=y_gdps  InternalRulePriority=Speed  RndMeth=Simplest  InputSameDT=on
  theta : Lookup_n-D  NumberOfTableDimensions=1  BreakpointsForDimension1=gradbp  Table=thetaRefab  InternalRulePriority=Speed  RndMeth=Simplest  InputSameDT=on
  refPose : Outport
  tag scope: Yaw_Ref=global, x_Ref=global, y_Ref=global
  wires:
  Integrator/1 -> X waypoints/1, theta/1, Y waypoints/1
  velFdk/1 -> Integrator/1
  Mux/1 -> refPose/1
  X waypoints/1 -> XY Graph/1, [x_Ref], Mux/1
  Y waypoints/1 -> [y_Ref], XY Graph/2, Mux/2
  theta/1 -> Mux/3, [Yaw_Ref]

== system MPC_Intersection_V2VandAIMandSTL/Vehicle 3D Dynamics/Powertrain & Driveline/Brake System ==
  Decc : Inport
  Hydraulics : autolibutils/Cont LPF  wc=30*pi*2  aMode=2
      settings: SourceProductBaseCode=PW,DR,MT,UV,VE
  Pressure : Gain  Gain=15e7
  Saturation1 : Saturate  UpperLimit=inf  LowerLimit=0  ZeroCross=off
  Selector : Selector  InputPortWidth=1  IndexOptions=Index vector (dialog)  Indices=[1 1 1 1]  OutputSizes=1
  Signal Specification : SignalSpecification  Unit=Pa
  Prs : Outport  PortDimensions=4  VectorParamsAs1DForOutWhenUnconnected=off
  wires:
  Signal Specification/1 -> Prs/1
  Decc/1 -> Saturation1/1
  Selector/1 -> Signal Specification/1
  Saturation1/1 -> Hydraulics/1
  Hydraulics/1 -> Pressure/1
  Pressure/1 -> Selector/1
